simulink model "open_loop_non_linear_model"  (R2019b)
settings: Solver=ode113  StartTime=0.0  StopTime=10  RelTol=1e-3
InitFcn:
  | addpath('generated');
  | cst = cellulo_constants();
  | 
  | c = cst.c;
  | c_U = cst.c_U;
settings Model: Creator=Hadrien  LastModifiedBy=Hadrien

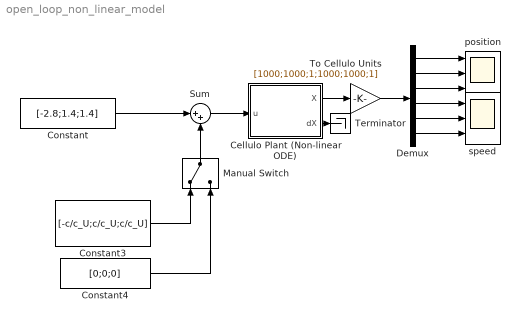
== system open_loop_non_linear_model ==
  Cellulo Plant (Non-linear ODE) : Subsystem
  Constant : Constant  Value=[-2.8;1.4;1.4]  VectorParams1D=off
  Constant3 : Constant  Value=[-c/c_U;c/c_U;c/c_U]  VectorParams1D=off
  Constant4 : Constant  Value=[0;0;0]  VectorParams1D=off
  Demux : Demux  Outputs=6
  Manual Switch : ManualSwitch
  Sum : Sum  Inputs=|++
  Terminator : Terminator
  To Cellulo Units : Gain  Gain=[1000;1000;1;1000;1000;1]
  position : Scope  NumInputPorts=3
  speed : Scope  NumInputPorts=3
  wires:
  Demux/6 -> speed/3
  Demux/5 -> speed/2
  Demux/4 -> speed/1
  Demux/2 -> position/2
  Demux/1 -> position/1
  Cellulo Plant (Non-linear ODE)/2(dX) -> Terminator/1
  Demux/3 -> position/3
  Cellulo Plant (Non-linear ODE)/1(X) -> To Cellulo Units/1
  To Cellulo Units/1 -> Demux/1
  Sum/1 -> Cellulo Plant (Non-linear ODE)/1(u)
  Manual Switch/1 -> Sum/2
  Constant3/1 -> Manual Switch/1
  Constant4/1 -> Manual Switch/2
  Constant/1 -> Sum/1

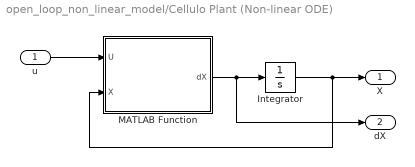
== system open_loop_non_linear_model/Cellulo Plant (Non-linear ODE) ==
  u : Inport  PortDimensions=3
  Integrator : Integrator
  MATLAB Function : MATLAB Function  TreatAsAtomicUnit=on
  X : Outport  PortDimensions=6
  dX : Outport  Port=2  PortDimensions=6
  wires:
  Integrator/1 -> X/1, MATLAB Function/2(X)
  u/1 -> MATLAB Function/1(U)
  MATLAB Function/1(dX) -> Integrator/1, dX/1

== matlab function open_loop_non_linear_model/Cellulo Plant (Non-linear ODE)/MATLAB Function ==
  data: U input; X input; dX output
function dX = Cellulo_ODE(U,X)

x = X(1);
y = X(2);
th = X(3);
dx = X(4);
dy = X(5);
dth = X(6);
u1 = U(1);
u2 = U(2);
u3 = U(3);

M = mass();
C = coriolis();
G = gravity();
D = friction(dth,dx,dy,th,u1,u2,u3);
Q = input_forces(th);
dq = reshape(X(4:6),3,1);
ddq = M\(-C*dq - G - D + Q*[u1;u2;u3]);
dX = [dq;ddq];
